simulink subsystem "processor"  (R2024b)
settings: Solver=VariableStepAuto  StartTime=0.0  StopTime=10.0  RelTol=1e-3
settings Model: Creator=finnb  LastModifiedBy=finnb

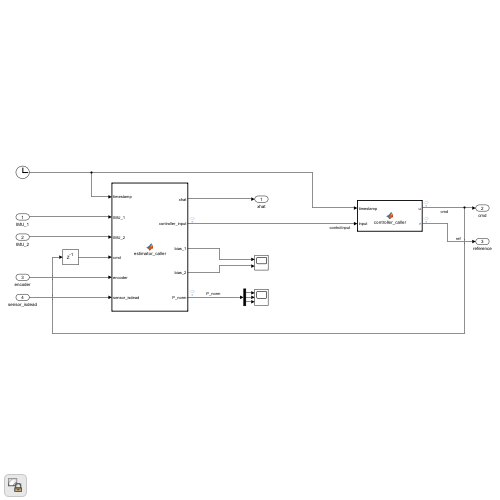
[thumbnail: Simulink's stored preview of the top-level diagram]
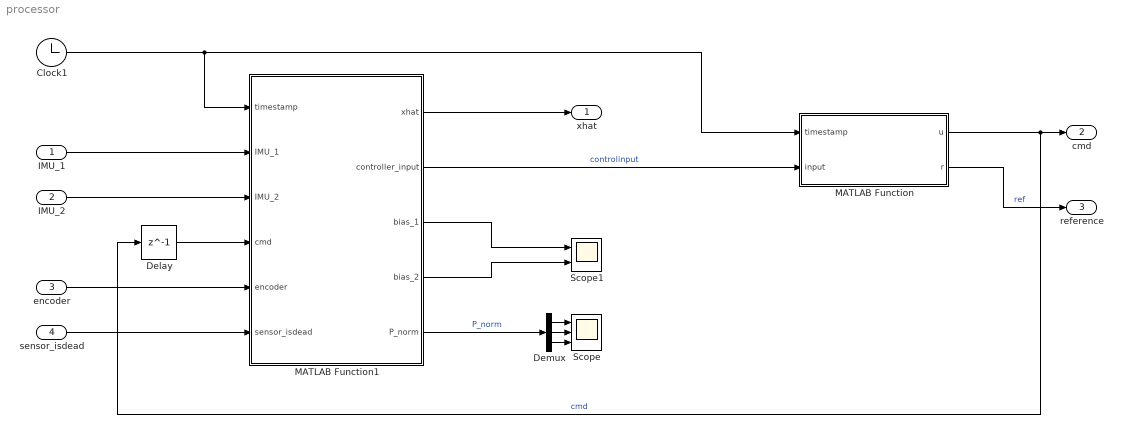
== system processor ==
  IMU_1 : Inport
  IMU_2 : Inport  Port=2
  encoder : Inport  Port=3
  sensor_isdead : Inport  Port=4
  Clock1 : Clock
  Delay : Delay  DelayLength=1
  Demux : Demux  Outputs=3
  MATLAB Function : MATLAB Function  TreatAsAtomicUnit=on
  MATLAB Function1 : MATLAB Function  TreatAsAtomicUnit=on
  Scope : Scope  NumInputPorts=3
  Scope1 : Scope  NumInputPorts=2
  xhat : Outport
  cmd : Outport  Port=2
  reference : Outport  Port=3
  wires:
  IMU_1/1 -> MATLAB Function1/2(IMU_1)
  Clock1/1 -> MATLAB Function/1(timestamp), MATLAB Function1/1(timestamp)
  IMU_2/1 -> MATLAB Function1/3(IMU_2)
  MATLAB Function1/1(xhat) -> xhat/1
  Delay/1 -> MATLAB Function1/4(cmd)
  encoder/1 -> MATLAB Function1/5(encoder)
  MATLAB Function1/5(P_norm) -> Demux/1  "P_norm"
  MATLAB Function1/4(bias_2) -> Scope1/2
  MATLAB Function1/3(bias_1) -> Scope1/1
  sensor_isdead/1 -> MATLAB Function1/6(sensor_isdead)
  Demux/1 -> Scope/1
  Demux/2 -> Scope/2
  Demux/3 -> Scope/3
  MATLAB Function/2(r) -> reference/1  "ref"
  MATLAB Function1/2(controller_input) -> MATLAB Function/2(input)  "controlinput"
  MATLAB Function/1(u) -> cmd/1, Delay/1  "cmd"

== matlab function processor/MATLAB Function ==
  settings: updateMethod=DISCRETE  sampleTime=samplingrate
  data: timestamp input size=1; input input size=5; u output size=1; r output
function [u, r] = controller_caller(timestamp, input)
    %#codegen
    u = 0;
    [u, r] = controller_module(timestamp, input);
end

== matlab function processor/MATLAB Function1 ==
  settings: updateMethod=DISCRETE  sampleTime=samplingrate
  data: timestamp input size=1; xhat output size=13; IMU_1 input size=10; IMU_2 input; cmd input size=1; encoder input size=1; controller_input output size=5; bias_1 output size=10; bias_2 output size=10; P_norm output size=3; sensor_isdead input
function [xhat, controller_input, bias_1, bias_2, P_norm] = estimator_caller(timestamp, IMU_1, IMU_2, cmd, encoder, sensor_isdead)

    % select IMUs, 1 is on, 0 is off, [IMU1, IMU2, encoder]
    sensor_select = [1; 1; 1]; 
    % sensor_select = cast(~sensor_isdead, 'double');

    IMU_1_handled = zeros(10,1);
    IMU_2_handled = zeros(10,1);
    [IMU_1_handled, IMU_2_handled] = imu_handler(IMU_1, IMU_2, sensor_select);
    % out = [IMU_1_handled(1:3), IMU_2_handled(1:3)];
    
    xhat = zeros(13,1);         
    Phat = zeros(13,13);
    controller_input = zeros(5,1);
    bias_1 = zeros(10,1);
    bias_2 = zeros(10,1);
    [xhat, Phat, controller_input, bias_1, bias_2] = estimator_module(timestamp, IMU_1_handled, IMU_2_handled, cmd, encoder, sensor_select);

    P_norm = zeros(3,1);
    P_norm = [det(Phat); cond(Phat); max([norm(Phat, 1), norm(Phat, 2), norm(Phat, Inf)])];
end
